simulink library "speblocks"  (Simulink 5.0)
libraries: simulink x1
settings Model: Creator=beryilma  LastModifiedBy=beryilma

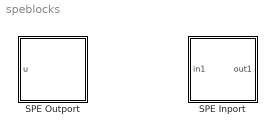
== system speblocks ==
  SPE Inport : Subsystem
      mask init:
      | st = 'SPE In';
      mask Display:
      | plot([0:0.1:1],[0 1. 0.55 0.90 0.65 0.80 0.7250 0.76 0.7450 0.75 0.75])
      | text(0.5, 0.4, st, 'HorizontalAlignment', 'center')
  SPE Outport : Subsystem  Tag=SPE_Out  mask(SPE Outport){}
      mask init:
      | st = 'SPE Out';
      settings: OpenFcn=disp('here')
      mask Display:
      | plot([0:0.1:1],[0 1. 0.55 0.90 0.65 0.80 0.7250 0.76 0.7450 0.75 0.75])
      | text(0.5, 0.4, st, 'HorizontalAlignment', 'center')

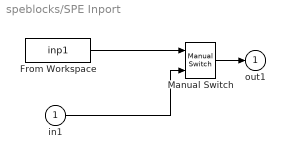
== system speblocks/SPE Inport ==
  in1 : Inport
  From Workspace : FromWorkspace  VariableName=inp1  SampleTime=0
  Manual Switch : simulink/Signal Routing/Manual Switch  sw=0  action=0
  out1 : Outport  InitialOutput=0
  wires:
  Manual Switch/1 -> out1/1
  in1/1 -> Manual Switch/2
  From Workspace/1 -> Manual Switch/1

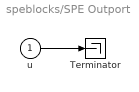
== system speblocks/SPE Outport ==
  u : Inport
  Terminator : Terminator
  wires:
  u/1 -> Terminator/1
